simulink model "CarSimROS"  (R2020b)
settings: Solver=FixedStepAuto  StartTime=0.0  StopTime=10.0  FixedStep=0.001  RelTol=1e-3
libraries: robotlib x13, simulink x1
(part 1 of 3)
settings Model: Creator=DwigHT  LastModifiedBy=DwigHT
settings OptimizationCC: EnhancedBackFolding=on  PassReuseOutputArgsAs=Individual arguments  ZeroExternalMemoryAtStartup=off  ZeroInternalMemoryAtStartup=off  MaxStackSize=64  OptimizeBlockOrder=speed  DifferentSizesBufferReuse=on  OptimizationCustomize=off  EfficientTunableParamExpr=on
settings DebuggingCC: ParameterTunabilityLossMsg=error
settings HardwareCC: ProdBitPerPointer=32  ProdBitPerSizeT=32  ProdBitPerPtrDiffT=32  ProdLargestAtomicFloat=None  ProdIntDivRoundTo=Undefined  ProdEndianess=Unspecified  ProdWordSize=32  ProdHWDeviceType=Generic->Unspecified (assume 32-bit Generic)
settings SFSimCC: MATLABDynamicMemAlloc=off
settings RTWCC: Description=Embedded Coder  SystemTargetFile=ert.tlc  HardwareBoard=Robot Operating System (ROS)  TLCOptions="-aInlineSetEventsForThisBaseRateFcn=TLC_FALSE -aSuppressMultiTaskScheduler=TLC_FALSE  -aRateBasedStepFcn=0"  TemplateMakefile=ert_default_tmf  Toolchain=Catkin  TargetLang=C++
settings CodeAppCC: ForceParamTrailComments=on  IgnoreCustomStorageClasses=off  OperatorAnnotations=on  SimulinkDataObjDesc=on  SFDataObjDesc=on  InsertBlockDesc=on
settings ERTTargetCC: SupportVariableSizeSignals=on

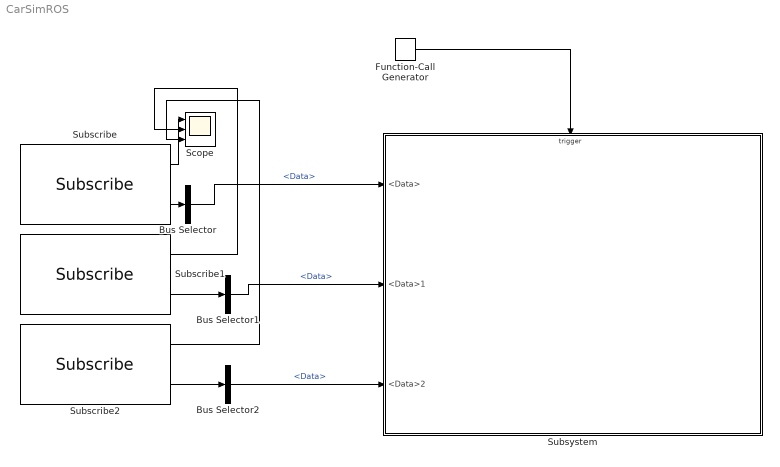
== system CarSimROS ==
  Bus Selector : BusSelector  OutputSignals=Data
  Bus Selector1 : BusSelector  OutputSignals=Data
  Bus Selector2 : BusSelector  OutputSignals=Data
  Function-Call Generator : simulink/Ports & Subsystems/Function-Call Generator  sample_time=0.1  numberOfIterations=1  DisallowWideOutput=off
  Scope : Scope  NumInputPorts=3
  Subscribe : robotlib/Subscribe  topicSource=Specify your own  topic=/Xr  messageType=std_msgs/Float64  SampleTime=-1  legacyBusStruct=off  messageQueueLength=1
  Subscribe1 : robotlib/Subscribe  topicSource=Specify your own  topic=/Yr  messageType=std_msgs/Float64  SampleTime=-1  legacyBusStruct=off  messageQueueLength=1
  Subscribe2 : robotlib/Subscribe  topicSource=Specify your own  topic=/Yaw  messageType=std_msgs/Float64  SampleTime=-1  legacyBusStruct=off  messageQueueLength=1
  Subsystem : Subsystem
  wires:
  Subscribe/2 -> Bus Selector/1
  Subscribe1/2 -> Bus Selector1/1
  Subscribe2/2 -> Bus Selector2/1
  Subscribe/1 -> Scope/1
  Subscribe1/1 -> Scope/2
  Subscribe2/1 -> Scope/3
  Bus Selector/1 -> Subsystem/1(<Data>)  "<Data>"
  Bus Selector1/1 -> Subsystem/2(<Data>1)  "<Data>"
  Bus Selector2/1 -> Subsystem/3(<Data>2)  "<Data>"
  Function-Call Generator/1 -> Subsystem/Trigger

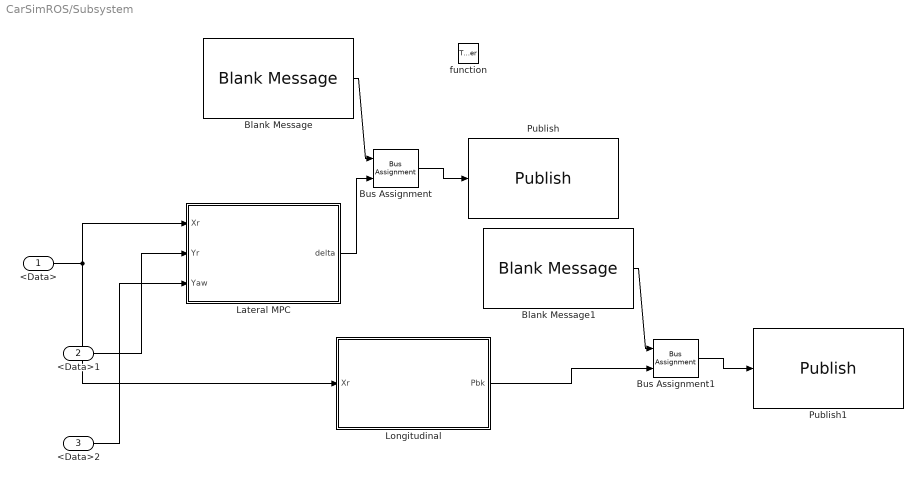
== system CarSimROS/Subsystem ==
  <Data> : Inport
  <Data>1 : Inport  Port=2
  <Data>2 : Inport  Port=3
  function : TriggerPort  TriggerType=function-call  VariantControl=Variant
  Blank Message : robotlib/Blank Message  messageClass=Message  entityType=std_msgs/Float64  messageType=std_msgs/Float64  SampleTime=inf  legacyBusStruct=off
  Blank Message1 : robotlib/Blank Message  messageClass=Message  entityType=std_msgs/Float64  messageType=std_msgs/Float64  SampleTime=inf  legacyBusStruct=off
  Bus Assignment : BusAssignment  AssignedSignals=Data
  Bus Assignment1 : BusAssignment  AssignedSignals=Data
  Lateral MPC : Subsystem
  Longitudinal : Subsystem
  Publish : robotlib/Publish  topicSource=Specify your own  topic=/delta  messageType=std_msgs/Float64  legacyBusStruct=off  messageQueueLength=1
  Publish1 : robotlib/Publish  topicSource=Specify your own  topic=/Pbk  messageType=std_msgs/Float64  legacyBusStruct=off  messageQueueLength=1
  wires:
  Bus Assignment/1 -> Publish/1
  Lateral MPC/1(delta) -> Bus Assignment/2
  Longitudinal/1(Pbk) -> Bus Assignment1/2
  <Data>/1 -> Lateral MPC/1(Xr), Longitudinal/1(Xr)
  Blank Message1/1 -> Bus Assignment1/1
  <Data>2/1 -> Lateral MPC/3(Yaw)
  Bus Assignment1/1 -> Publish1/1
  Blank Message/1 -> Bus Assignment/1
  <Data>1/1 -> Lateral MPC/2(Yr)

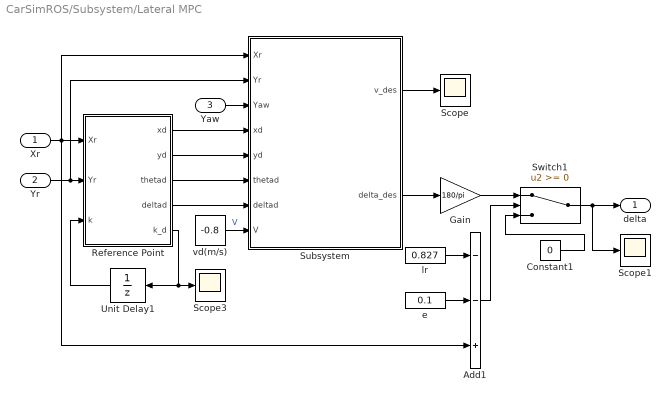
== system CarSimROS/Subsystem/Lateral MPC ==
  Xr : Inport
  Yr : Inport  Port=2
  Yaw : Inport  Port=3
  Add1 : Sum  Inputs=--+
  Constant1 : Constant  Value=0
  Gain : Gain  Gain=180/pi
  Reference Point : MATLAB Function  TreatAsAtomicUnit=on
  Scope : Scope
  Scope1 : Scope
  Scope3 : Scope
  Subsystem : Subsystem
  Switch1 : Switch
  Unit Delay1 : UnitDelay  InitialCondition=1  SampleTime=-1  HasFrameUpgradeWarning=on
  e : Constant  Value=0.1
  lr : Constant  Value=0.827
  vd(m/s) : Constant  Value=-0.8
  delta : Outport  VectorParamsAs1DForOutWhenUnconnected=off
  wires:
  Reference Point/2(yd) -> Subsystem/5(yd)
  vd(m/s)/1 -> Subsystem/8(V)  "V"
  Reference Point/4(deltad) -> Subsystem/7(deltad)
  Reference Point/3(thetad) -> Subsystem/6(thetad)
  Unit Delay1/1 -> Reference Point/3(k)
  Reference Point/1(xd) -> Subsystem/4(xd)
  Reference Point/5(k_d) -> Scope3/1, Unit Delay1/1
  Switch1/1 -> Scope1/1, delta/1
  Gain/1 -> Switch1/1
  Yr/1 -> Subsystem/2(Yr), Reference Point/2(Yr)
  Yaw/1 -> Subsystem/3(Yaw)
  Subsystem/1(v_des) -> Scope/1
  Subsystem/2(delta_des) -> Gain/1
  e/1 -> Add1/2
  lr/1 -> Add1/1
  Constant1/1 -> Switch1/3
  Add1/1 -> Switch1/2
  Xr/1 -> Add1/3, Subsystem/1(Xr), Reference Point/1(Xr)

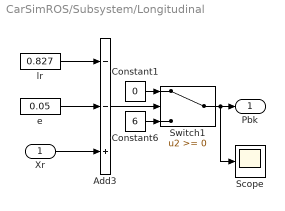
== system CarSimROS/Subsystem/Longitudinal ==
  Xr : Inport
  Add3 : Sum  Inputs=--+
  Constant1 : Constant  Value=0
  Constant6 : Constant  Value=6
  Scope : Scope
  Switch1 : Switch
  e : Constant  Value=0.05
  lr : Constant  Value=0.827
  Pbk : Outport  VectorParamsAs1DForOutWhenUnconnected=off
  wires:
  Constant6/1 -> Switch1/3
  Add3/1 -> Switch1/2
  Xr/1 -> Add3/3
  e/1 -> Add3/2
  lr/1 -> Add3/1
  Constant1/1 -> Switch1/1
  Switch1/1 -> Scope/1, Pbk/1

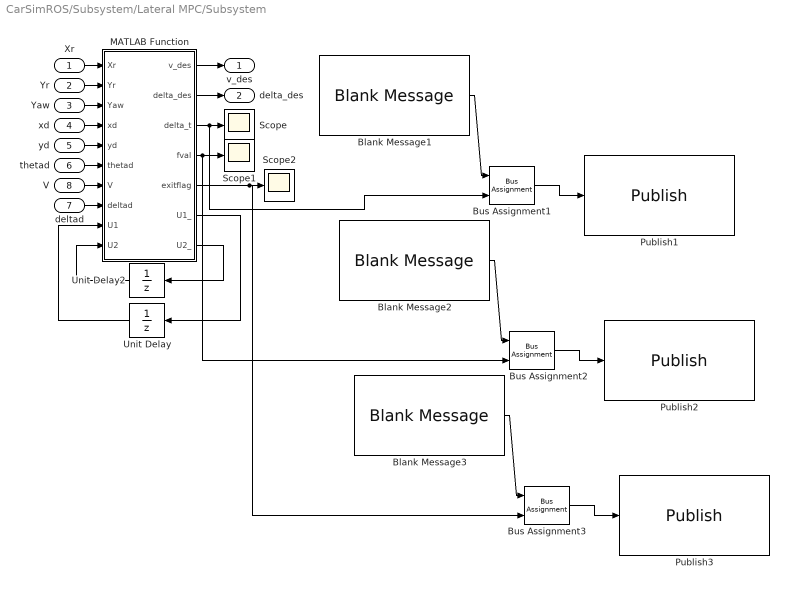
== system CarSimROS/Subsystem/Lateral MPC/Subsystem ==
  Xr : Inport
  Yr : Inport  Port=2
  Yaw : Inport  Port=3
  xd : Inport  Port=4
  yd : Inport  Port=5
  thetad : Inport  Port=6
  deltad : Inport  Port=7
  V : Inport  Port=8
  Blank Message1 : robotlib/Blank Message  messageClass=Message  entityType=std_msgs/Float64  messageType=std_msgs/Float64  SampleTime=inf  legacyBusStruct=off
  Blank Message2 : robotlib/Blank Message  messageClass=Message  entityType=std_msgs/Float64  messageType=std_msgs/Float64  SampleTime=inf  legacyBusStruct=off
  Blank Message3 : robotlib/Blank Message  messageClass=Message  entityType=std_msgs/Float64  messageType=std_msgs/Float64  SampleTime=inf  legacyBusStruct=off
  Bus Assignment1 : BusAssignment  AssignedSignals=Data
  Bus Assignment2 : BusAssignment  AssignedSignals=Data
  Bus Assignment3 : BusAssignment  AssignedSignals=Data
  MATLAB Function : MATLAB Function  TreatAsAtomicUnit=on
  Publish1 : robotlib/Publish  topicSource=Specify your own  topic=/delta_t  messageType=std_msgs/Float64  legacyBusStruct=off  messageQueueLength=1
  Publish2 : robotlib/Publish  topicSource=Specify your own  topic=/fval  messageType=std_msgs/Float64  legacyBusStruct=off  messageQueueLength=1
  Publish3 : robotlib/Publish  topicSource=Specify your own  topic=/exitflag  messageType=std_msgs/Float64  legacyBusStruct=off  messageQueueLength=1
  Scope : Scope
  Scope1 : Scope
  Scope2 : Scope
  Unit Delay : UnitDelay  SampleTime=-1  HasFrameUpgradeWarning=on
  Unit Delay2 : UnitDelay  SampleTime=-1  HasFrameUpgradeWarning=on
  v_des : Outport
  delta_des : Outport  Port=2
  wires:
  Unit Delay/1 -> MATLAB Function/9(U1)
  MATLAB Function/7(U2_) -> Unit Delay2/1
  Unit Delay2/1 -> MATLAB Function/10(U2)
  Yr/1 -> MATLAB Function/2(Yr)
  yd/1 -> MATLAB Function/5(yd)
  MATLAB Function/6(U1_) -> Unit Delay/1
  MATLAB Function/5(exitflag) -> Bus Assignment3/2, Scope2/1
  xd/1 -> MATLAB Function/4(xd)
  V/1 -> MATLAB Function/7(V)
  MATLAB Function/1(v_des) -> v_des/1
  Xr/1 -> MATLAB Function/1(Xr)
  Yaw/1 -> MATLAB Function/3(Yaw)
  thetad/1 -> MATLAB Function/6(thetad)
  MATLAB Function/2(delta_des) -> delta_des/1
  deltad/1 -> MATLAB Function/8(deltad)
  Bus Assignment1/1 -> Publish1/1
  Blank Message1/1 -> Bus Assignment1/1
  MATLAB Function/4(fval) -> Scope1/1, Bus Assignment2/2
  Blank Message2/1 -> Bus Assignment2/1
  Bus Assignment2/1 -> Publish2/1
  Bus Assignment3/1 -> Publish3/1
  Blank Message3/1 -> Bus Assignment3/1
  MATLAB Function/3(delta_t) -> Bus Assignment1/2, Scope/1
